simulink model "FOPTD_model_simulink"  (R2020a)
settings: Solver=FixedStepAuto  StartTime=0.0  StopTime=600  FixedStep=1  RelTol=1e-3
values from neighbouring files (symbols this model uses):
  K = x(1)    [FOPTD_model_PSO_method.m]    (also in FOPTD_model_plot.m = 0.7243; FOPTD_model_twopoint_method.m = (y_final - y_initial)/(u_final - u_initial))
  L = x(3)    [FOPTD_model_PSO_method.m]    (also in FOPTD_model_plot.m = 33.398; FOPTD_model_twopoint_method.m = 1.3*(y_35_time - TIME_STEP) - 0.29*(y_85_time - TIME_STEP))
  T = x(2)    [FOPTD_model_PSO_method.m]    (also in FOPTD_model_plot.m = 162.4602; FOPTD_model_twopoint_method.m = 0.67*((y_85_time - TIME_STEP) - (y_35_time - TIME_STEP)))
  y_initial = TCLab_data.T1(TIME_STEP)    [FOPTD_model_PSO_method.m]    (also in FOPTD_model_plot.m; FOPTD_model_twopoint_method.m)
settings Model: Creator=itsri  LastModifiedBy=pedro_000
settings DataIOCC: ReturnWorkspaceOutputs=off

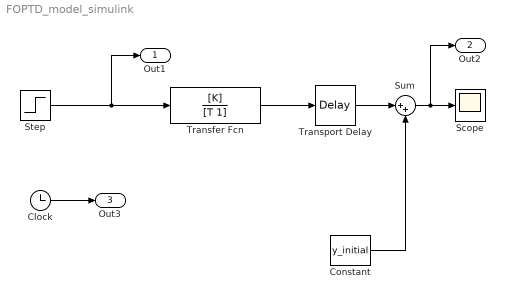
== system FOPTD_model_simulink ==
  Clock : Clock
  Constant : Constant  Value=y_initial
  Scope : Scope
  Step : Step  After=80  SampleTime=0
  Sum : Sum  Inputs=|++
  Transfer Fcn : TransferFcn  Numerator=[K]  Denominator=[T 1]
  Transport Delay : TransportDelay  DelayTime=L
  Out1 : Outport  SampleTime=1
  Out2 : Outport  Port=2  SampleTime=1
  Out3 : Outport  Port=3  SampleTime=1
  wires:
  Clock/1 -> Out3/1
  Transfer Fcn/1 -> Transport Delay/1
  Step/1 -> Transfer Fcn/1, Out1/1
  Sum/1 -> Out2/1, Scope/1
  Transport Delay/1 -> Sum/1
  Constant/1 -> Sum/2
